simulink model "model_InputConditioningAutoRestart"  (R2024a)
settings: Solver=FixedStepAuto  StartTime=0.0  StopTime=10.0  RelTol=1e-3
settings Model: Creator=Gabriel  LastModifiedBy=Gabriel

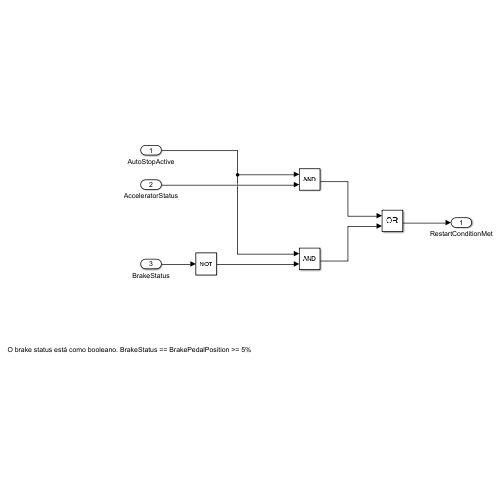
[thumbnail: Simulink's stored preview of the top-level diagram]
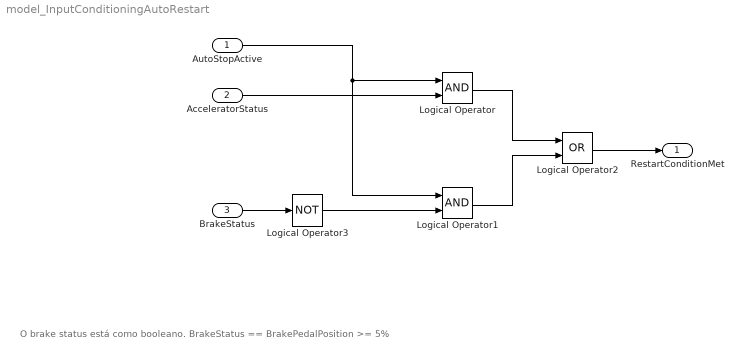
== system model_InputConditioningAutoRestart ==
  note: O brake status está como booleano. BrakeStatus == BrakePedalPosition >= 5%
  AutoStopActive : Inport
  AcceleratorStatus : Inport  Port=2
  BrakeStatus : Inport  Port=3
  Logical Operator : Logic  AllPortsSameDT=off  OutDataTypeStr=boolean
  Logical Operator1 : Logic  AllPortsSameDT=off  OutDataTypeStr=boolean
  Logical Operator2 : Logic  Operator=OR  AllPortsSameDT=off  OutDataTypeStr=boolean
  Logical Operator3 : Logic  Operator=NOT  AllPortsSameDT=off  OutDataTypeStr=boolean
  RestartConditionMet : Outport
  wires:
  Logical Operator3/1 -> Logical Operator1/2
  Logical Operator2/1 -> RestartConditionMet/1
  AutoStopActive/1 -> Logical Operator1/1, Logical Operator/1
  Logical Operator/1 -> Logical Operator2/1
  Logical Operator1/1 -> Logical Operator2/2
  BrakeStatus/1 -> Logical Operator3/1
  AcceleratorStatus/1 -> Logical Operator/2
